simulink model "Model"  (R2023b)
settings: Solver=FixedStepAuto  StartTime=0.0  StopTime=10  FixedStep=0.002  RelTol=1e-3
model workspace (MAT data in the model file):
  a = 0
undefined symbols (not defined in the file or in its folder): X, Y, Z
libraries: sm_lib x84, nesl_utility x29, slpidlib x9, simulink x6
(part 7 of 7)

== matlab function Model/支持力结算/MATLAB Function2 ==
  data: m_w input; F_N output; T1 input; T2 input; a_w input; theta input; phi_1 input; phi_4 input; L_0 input
function F_N = fcn(m_w,T1,T2,a_w,theta,phi_1,phi_4,L_0)

l_1=0.15;
l_2=0.27;
l_3=0.27;
l_4=0.15;
l_5=0.15;g=9.80665;

J11=(2*(l_1*cos(phi_1) + (2*l_2*cos(2*atan(((4*l_2^2*(l_1*sin(phi_1) - l_4*sin(phi_4))^2 - ((l_1*sin(phi_1) - l_4*sin(phi_4))^2 + (l_5 - l_1*cos(phi_1) + l_4*cos(phi_4))^2 + l_2^2 - l_3^2)^2 + 4*l_2^2*(l_5 - l_1*cos(phi_1) + l_4*cos(phi_4))^2)^(1/2) - 2*l_2*(l_1*sin(phi_1) - l_4*sin(phi_4)))/((l_1*sin(phi_1) - l_4*sin(phi_4))^2 + (l_5 - l_1*cos(phi_1) + l_4*cos(phi_4))^2 + l_2^2 - l_3^2 + 2*l_2*(l_5 - l_1*cos(phi_1) + l_4*cos(phi_4)))))*(((8*l_1*l_2^2*cos(phi_1)*(l_1*sin(phi_1) - l_4*sin(phi_4)) - 2*(2*l_1*cos(phi_1)*(l_1*sin(phi_1) - l_4*sin(phi_4)) + 2*l_1*sin(phi_1)*(l_5 - l_1*cos(phi_1) + l_4*cos(phi_4)))*((l_1*sin(phi_1) - l_4*sin(phi_4))^2 + (l_5 - l_1*cos(phi_1) + l_4*cos(phi_4))^2 + l_2^2 - l_3^2) + 8*l_1*l_2^2*sin(phi_1)*(l_5 - l_1*cos(phi_1) + l_4*cos(phi_4)))/(2*(4*l_2^2*(l_1*sin(phi_1) - l_4*sin(phi_4))^2 - ((l_1*sin(phi_1) - l_4*sin(phi_4))^2 + (l_5 - l_1*cos(phi_1) + l_4*cos(phi_4))^2 + l_2^2 - l_3^2)^2 + 4*l_2^2*(l_5 - l_1*cos(phi_1) + l_4*cos(phi_4))^2)^(1/2)) - 2*l_1*l_2*cos(phi_1))/((l_1*sin(phi_1) - l_4*sin(phi_4))^2 + (l_5 - l_1*cos(phi_1) + l_4*cos(phi_4))^2 + l_2^2 - l_3^2 + 2*l_2*(l_5 - l_1*cos(phi_1) + l_4*cos(phi_4))) - (((4*l_2^2*(l_1*sin(phi_1) - l_4*sin(phi_4))^2 - ((l_1*sin(phi_1) - l_4*sin(phi_4))^2 + (l_5 - l_1*cos(phi_1) + l_4*cos(phi_4))^2 + l_2^2 - l_3^2)^2 + 4*l_2^2*(l_5 - l_1*cos(phi_1) + l_4*cos(phi_4))^2)^(1/2) - 2*l_2*(l_1*sin(phi_1) - l_4*sin(phi_4)))*(2*l_1*l_2*sin(phi_1) + 2*l_1*cos(phi_1)*(l_1*sin(phi_1) - l_4*sin(phi_4)) + 2*l_1*sin(phi_1)*(l_5 - l_1*cos(phi_1) + l_4*cos(phi_4))))/((l_1*sin(phi_1) - l_4*sin(phi_4))^2 + (l_5 - l_1*cos(phi_1) + l_4*cos(phi_4))^2 + l_2^2 - l_3^2 + 2*l_2*(l_5 - l_1*cos(phi_1) + l_4*cos(phi_4)))^2))/(((4*l_2^2*(l_1*sin(phi_1) - l_4*sin(phi_4))^2 - ((l_1*sin(phi_1) - l_4*sin(phi_4))^2 + (l_5 - l_1*cos(phi_1) + l_4*cos(phi_4))^2 + l_2^2 - l_3^2)^2 + 4*l_2^2*(l_5 - l_1*cos(phi_1) + l_4*cos(phi_4))^2)^(1/2) - 2*l_2*(l_1*sin(phi_1) - l_4*sin(phi_4)))^2/((l_1*sin(phi_1) - l_4*sin(phi_4))^2 + (l_5 - l_1*cos(phi_1) + l_4*cos(phi_4))^2 + l_2^2 - l_3^2 + 2*l_2*(l_5 - l_1*cos(phi_1) + l_4*cos(phi_4)))^2 + 1))*(l_2*sin(2*atan(((4*l_2^2*(l_1*sin(phi_1) - l_4*sin(phi_4))^2 - ((l_1*sin(phi_1) - l_4*sin(phi_4))^2 + (l_5 - l_1*cos(phi_1) + l_4*cos(phi_4))^2 + l_2^2 - l_3^2)^2 + 4*l_2^2*(l_5 - l_1*cos(phi_1) + l_4*cos(phi_4))^2)^(1/2) - 2*l_2*(l_1*sin(phi_1) - l_4*sin(phi_4)))/((l_1*sin(phi_1) - l_4*sin(phi_4))^2 + (l_5 - l_1*cos(phi_1) + l_4*cos(phi_4))^2 + l_2^2 - l_3^2 + 2*l_2*(l_5 - l_1*cos(phi_1) + l_4*cos(phi_4))))) + l_1*sin(phi_1)) - 2*(l_1*sin(phi_1) + (2*l_2*sin(2*atan(((4*l_2^2*(l_1*sin(phi_1) - l_4*sin(phi_4))^2 - ((l_1*sin(phi_1) - l_4*sin(phi_4))^2 + (l_5 - l_1*cos(phi_1) + l_4*cos(phi_4))^2 + l_2^2 - l_3^2)^2 + 4*l_2^2*(l_5 - l_1*cos(phi_1) + l_4*cos(phi_4))^2)^(1/2) - 2*l_2*(l_1*sin(phi_1) - l_4*sin(phi_4)))/((l_1*sin(phi_1) - l_4*sin(phi_4))^2 + (l_5 - l_1*cos(phi_1) + l_4*cos(phi_4))^2 + l_2^2 - l_3^2 + 2*l_2*(l_5 - l_1*cos(phi_1) + l_4*cos(phi_4)))))*(((8*l_1*l_2^2*cos(phi_1)*(l_1*sin(phi_1) - l_4*sin(phi_4)) - 2*(2*l_1*cos(phi_1)*(l_1*sin(phi_1) - l_4*sin(phi_4)) + 2*l_1*sin(phi_1)*(l_5 - l_1*cos(phi_1) + l_4*cos(phi_4)))*((l_1*sin(phi_1) - l_4*sin(phi_4))^2 + (l_5 - l_1*cos(phi_1) + l_4*cos(phi_4))^2 + l_2^2 - l_3^2) + 8*l_1*l_2^2*sin(phi_1)*(l_5 - l_1*cos(phi_1) + l_4*cos(phi_4)))/(2*(4*l_2^2*(l_1*sin(phi_1) - l_4*sin(phi_4))^2 - ((l_1*sin(phi_1) - l_4*sin(phi_4))^2 + (l_5 - l_1*cos(phi_1) + l_4*cos(phi_4))^2 + l_2^2 - l_3^2)^2 + 4*l_2^2*(l_5 - l_1*cos(phi_1) + l_4*cos(phi_4))^2)^(1/2)) - 2*l_1*l_2*cos(phi_1))/((l_1*sin(phi_1) - l_4*sin(phi_4))^2 + (l_5 - l_1*cos(phi_1) + l_4*cos(phi_4))^2 + l_2^2 - l_3^2 + 2*l_2*(l_5 - l_1*cos(phi_1) + l_4*cos(phi_4))) - (((4*l_2^2*(l_1*sin(phi_1) - l_4*sin(phi_4))^2 - ((l_1*sin(phi_1) - l_4*sin(phi_4))^2 + (l_5 - l_1*cos(phi_1) + l_4*cos(phi_4))^2 + l_2^2 - l_3^2)^2 + 4*l_2^2*(l_5 - l_1*cos(phi_1) + l_4*cos(phi_4))^2)^(1/2) - 2*l_2*(l_1*sin(phi_1) - l_4*sin(phi_4)))*(2*l_1*l_2*sin(phi_1) + 2*l_1*cos(phi_1)*(l_1*sin(phi_1) - l_4*sin(phi_4)) + 2*l_1*sin(phi_1)*(l_5 - l_1*cos(phi_1) + l_4*cos(phi_4))))/((l_1*sin(phi_1) - l_4*sin(phi_4))^2 + (l_5 - l_1*cos(phi_1) + l_4*cos(phi_4))^2 + l_2^2 - l_3^2 + 2*l_2*(l_5 - l_1*cos(phi_1) + l_4*cos(phi_4)))^2))/(((4*l_2^2*(l_1*sin(phi_1) - l_4*sin(phi_4))^2 - ((l_1*sin(phi_1) - l_4*sin(phi_4))^2 + (l_5 - l_1*cos(phi_1) + l_4*cos(phi_4))^2 + l_2^2 - l_3^2)^2 + 4*l_2^2*(l_5 - l_1*cos(phi_1) + l_4*cos(phi_4))^2)^(1/2) - 2*l_2*(l_1*sin(phi_1) - l_4*sin(phi_4)))^2/((l_1*sin(phi_1) - l_4*sin(phi_4))^2 + (l_5 - l_1*cos(phi_1) + l_4*cos(phi_4))^2 + l_2^2 - l_3^2 + 2*l_2*(l_5 - l_1*cos(phi_1) + l_4*cos(phi_4)))^2 + 1))*(l_2*cos(2*atan(((4*l_2^2*(l_1*sin(phi_1) - l_4*sin(phi_4))^2 - ((l_1*sin(phi_1) - l_4*sin(phi_4))^2 + (l_5 - l_1*cos(phi_1) + l_4*cos(phi_4))^2 + l_2^2 - l_3^2)^2 + 4*l_2^2*(l_5 - l_1*cos(phi_1) + l_4*cos(phi_4))^2)^(1/2) - 2*l_2*(l_1*sin(phi_1) - l_4*sin(phi_4)))/((l_1*sin(phi_1) - l_4*sin(phi_4))^2 + (l_5 - l_1*cos(phi_1) + l_4*cos(phi_4))^2 + l_2^2 - l_3^2 + 2*l_2*(l_5 - l_1*cos(phi_1) + l_4*cos(phi_4))))) - l_5/2 + l_1*cos(phi_1)))/(2*((l_2*sin(2*atan(((4*l_2^2*(l_1*sin(phi_1) - l_4*sin(phi_4))^2 - ((l_1*sin(phi_1) - l_4*sin(phi_4))^2 + (l_5 - l_1*cos(phi_1) + l_4*cos(phi_4))^2 + l_2^2 - l_3^2)^2 + 4*l_2^2*(l_5 - l_1*cos(phi_1) + l_4*cos(phi_4))^2)^(1/2) - 2*l_2*(l_1*sin(phi_1) - l_4*sin(phi_4)))/((l_1*sin(phi_1) - l_4*sin(phi_4))^2 + (l_5 - l_1*cos(phi_1) + l_4*cos(phi_4))^2 + l_2^2 - l_3^2 + 2*l_2*(l_5 - l_1*cos(phi_1) + l_4*cos(phi_4))))) + l_1*sin(phi_1))^2 + (l_2*cos(2*atan(((4*l_2^2*(l_1*sin(phi_1) - l_4*sin(phi_4))^2 - ((l_1*sin(phi_1) - l_4*sin(phi_4))^2 + (l_5 - l_1*cos(phi_1) + l_4*cos(phi_4))^2 + l_2^2 - l_3^2)^2 + 4*l_2^2*(l_5 - l_1*cos(phi_1) + l_4*cos(phi_4))^2)^(1/2) - 2*l_2*(l_1*sin(phi_1) - l_4*sin(phi_4)))/((l_1*sin(phi_1) - l_4*sin(phi_4))^2 + (l_5 - l_1*cos(phi_1) + l_4*cos(phi_4))^2 + l_2^2 - l_3^2 + 2*l_2*(l_5 - l_1*cos(phi_1) + l_4*cos(phi_4))))) - l_5/2 + l_1*cos(phi_1))^2)^(1/2));
J12=((4*l_2*sin(2*atan(((4*l_2^2*(l_1*sin(phi_1) - l_4*sin(phi_4))^2 - ((l_1*sin(phi_1) - l_4*sin(phi_4))^2 + (l_5 - l_1*cos(phi_1) + l_4*cos(phi_4))^2 + l_2^2 - l_3^2)^2 + 4*l_2^2*(l_5 - l_1*cos(phi_1) + l_4*cos(phi_4))^2)^(1/2) - 2*l_2*(l_1*sin(phi_1) - l_4*sin(phi_4)))/((l_1*sin(phi_1) - l_4*sin(phi_4))^2 + (l_5 - l_1*cos(phi_1) + l_4*cos(phi_4))^2 + l_2^2 - l_3^2 + 2*l_2*(l_5 - l_1*cos(phi_1) + l_4*cos(phi_4)))))*(((8*l_2^2*l_4*cos(phi_4)*(l_1*sin(phi_1) - l_4*sin(phi_4)) - 2*(2*l_4*cos(phi_4)*(l_1*sin(phi_1) - l_4*sin(phi_4)) + 2*l_4*sin(phi_4)*(l_5 - l_1*cos(phi_1) + l_4*cos(phi_4)))*((l_1*sin(phi_1) - l_4*sin(phi_4))^2 + (l_5 - l_1*cos(phi_1) + l_4*cos(phi_4))^2 + l_2^2 - l_3^2) + 8*l_2^2*l_4*sin(phi_4)*(l_5 - l_1*cos(phi_1) + l_4*cos(phi_4)))/(2*(4*l_2^2*(l_1*sin(phi_1) - l_4*sin(phi_4))^2 - ((l_1*sin(phi_1) - l_4*sin(phi_4))^2 + (l_5 - l_1*cos(phi_1) + l_4*cos(phi_4))^2 + l_2^2 - l_3^2)^2 + 4*l_2^2*(l_5 - l_1*cos(phi_1) + l_4*cos(phi_4))^2)^(1/2)) - 2*l_2*l_4*cos(phi_4))/((l_1*sin(phi_1) - l_4*sin(phi_4))^2 + (l_5 - l_1*cos(phi_1) + l_4*cos(phi_4))^2 + l_2^2 - l_3^2 + 2*l_2*(l_5 - l_1*cos(phi_1) + l_4*cos(phi_4))) - (((4*l_2^2*(l_1*sin(phi_1) - l_4*sin(phi_4))^2 - ((l_1*sin(phi_1) - l_4*sin(phi_4))^2 + (l_5 - l_1*cos(phi_1) + l_4*cos(phi_4))^2 + l_2^2 - l_3^2)^2 + 4*l_2^2*(l_5 - l_1*cos(phi_1) + l_4*cos(phi_4))^2)^(1/2) - 2*l_2*(l_1*sin(phi_1) - l_4*sin(phi_4)))*(2*l_2*l_4*sin(phi_4) + 2*l_4*cos(phi_4)*(l_1*sin(phi_1) - l_4*sin(phi_4)) + 2*l_4*sin(phi_4)*(l_5 - l_1*cos(phi_1) + l_4*cos(phi_4))))/((l_1*sin(phi_1) - l_4*sin(phi_4))^2 + (l_5 - l_1*cos(phi_1) + l_4*cos(phi_4))^2 + l_2^2 - l_3^2 + 2*l_2*(l_5 - l_1*cos(phi_1) + l_4*cos(phi_4)))^2)*(l_2*cos(2*atan(((4*l_2^2*(l_1*sin(phi_1) - l_4*sin(phi_4))^2 - ((l_1*sin(phi_1) - l_4*sin(phi_4))^2 + (l_5 - l_1*cos(phi_1) + l_4*cos(phi_4))^2 + l_2^2 - l_3^2)^2 + 4*l_2^2*(l_5 - l_1*cos(phi_1) + l_4*cos(phi_4))^2)^(1/2) - 2*l_2*(l_1*sin(phi_1) - l_4*sin(phi_4)))/((l_1*sin(phi_1) - l_4*sin(phi_4))^2 + (l_5 - l_1*cos(phi_1) + l_4*cos(phi_4))^2 + l_2^2 - l_3^2 + 2*l_2*(l_5 - l_1*cos(phi_1) + l_4*cos(phi_4))))) - l_5/2 + l_1*cos(phi_1)))/(((4*l_2^2*(l_1*sin(phi_1) - l_4*sin(phi_4))^2 - ((l_1*sin(phi_1) - l_4*sin(phi_4))^2 + (l_5 - l_1*cos(phi_1) + l_4*cos(phi_4))^2 + l_2^2 - l_3^2)^2 + 4*l_2^2*(l_5 - l_1*cos(phi_1) + l_4*cos(phi_4))^2)^(1/2) - 2*l_2*(l_1*sin(phi_1) - l_4*sin(phi_4)))^2/((l_1*sin(phi_1) - l_4*sin(phi_4))^2 + (l_5 - l_1*cos(phi_1) + l_4*cos(phi_4))^2 + l_2^2 - l_3^2 + 2*l_2*(l_5 - l_1*cos(phi_1) + l_4*cos(phi_4)))^2 + 1) - (4*l_2*cos(2*atan(((4*l_2^2*(l_1*sin(phi_1) - l_4*sin(phi_4))^2 - ((l_1*sin(phi_1) - l_4*sin(phi_4))^2 + (l_5 - l_1*cos(phi_1) + l_4*cos(phi_4))^2 + l_2^2 - l_3^2)^2 + 4*l_2^2*(l_5 - l_1*cos(phi_1) + l_4*cos(phi_4))^2)^(1/2) - 2*l_2*(l_1*sin(phi_1) - l_4*sin(phi_4)))/((l_1*sin(phi_1) - l_4*sin(phi_4))^2 + (l_5 - l_1*cos(phi_1) + l_4*cos(phi_4))^2 + l_2^2 - l_3^2 + 2*l_2*(l_5 - l_1*cos(phi_1) + l_4*cos(phi_4)))))*(l_2*sin(2*atan(((4*l_2^2*(l_1*sin(phi_1) - l_4*sin(phi_4))^2 - ((l_1*sin(phi_1) - l_4*sin(phi_4))^2 + (l_5 - l_1*cos(phi_1) + l_4*cos(phi_4))^2 + l_2^2 - l_3^2)^2 + 4*l_2^2*(l_5 - l_1*cos(phi_1) + l_4*cos(phi_4))^2)^(1/2) - 2*l_2*(l_1*sin(phi_1) - l_4*sin(phi_4)))/((l_1*sin(phi_1) - l_4*sin(phi_4))^2 + (l_5 - l_1*cos(phi_1) + l_4*cos(phi_4))^2 + l_2^2 - l_3^2 + 2*l_2*(l_5 - l_1*cos(phi_1) + l_4*cos(phi_4))))) + l_1*sin(phi_1))*(((8*l_2^2*l_4*cos(phi_4)*(l_1*sin(phi_1) - l_4*sin(phi_4)) - 2*(2*l_4*cos(phi_4)*(l_1*sin(phi_1) - l_4*sin(phi_4)) + 2*l_4*sin(phi_4)*(l_5 - l_1*cos(phi_1) + l_4*cos(phi_4)))*((l_1*sin(phi_1) - l_4*sin(phi_4))^2 + (l_5 - l_1*cos(phi_1) + l_4*cos(phi_4))^2 + l_2^2 - l_3^2) + 8*l_2^2*l_4*sin(phi_4)*(l_5 - l_1*cos(phi_1) + l_4*cos(phi_4)))/(2*(4*l_2^2*(l_1*sin(phi_1) - l_4*sin(phi_4))^2 - ((l_1*sin(phi_1) - l_4*sin(phi_4))^2 + (l_5 - l_1*cos(phi_1) + l_4*cos(phi_4))^2 + l_2^2 - l_3^2)^2 + 4*l_2^2*(l_5 - l_1*cos(phi_1) + l_4*cos(phi_4))^2)^(1/2)) - 2*l_2*l_4*cos(phi_4))/((l_1*sin(phi_1) - l_4*sin(phi_4))^2 + (l_5 - l_1*cos(phi_1) + l_4*cos(phi_4))^2 + l_2^2 - l_3^2 + 2*l_2*(l_5 - l_1*cos(phi_1) + l_4*cos(phi_4))) - (((4*l_2^2*(l_1*sin(phi_1) - l_4*sin(phi_4))^2 - ((l_1*sin(phi_1) - l_4*sin(phi_4))^2 + (l_5 - l_1*cos(phi_1) + l_4*cos(phi_4))^2 + l_2^2 - l_3^2)^2 + 4*l_2^2*(l_5 - l_1*cos(phi_1) + l_4*cos(phi_4))^2)^(1/2) - 2*l_2*(l_1*sin(phi_1) - l_4*sin(phi_4)))*(2*l_2*l_4*sin(phi_4) + 2*l_4*cos(phi_4)*(l_1*sin(phi_1) - l_4*sin(phi_4)) + 2*l_4*sin(phi_4)*(l_5 - l_1*cos(phi_1) + l_4*cos(phi_4))))/((l_1*sin(phi_1) - l_4*sin(phi_4))^2 + (l_5 - l_1*cos(phi_1) + l_4*cos(phi_4))^2 + l_2^2 - l_3^2 + 2*l_2*(l_5 - l_1*cos(phi_1) + l_4*cos(phi_4)))^2))/(((4*l_2^2*(l_1*sin(phi_1) - l_4*sin(phi_4))^2 - ((l_1*sin(phi_1) - l_4*sin(phi_4))^2 + (l_5 - l_1*cos(phi_1) + l_4*cos(phi_4))^2 + l_2^2 - l_3^2)^2 + 4*l_2^2*(l_5 - l_1*cos(phi_1) + l_4*cos(phi_4))^2)^(1/2) - 2*l_2*(l_1*sin(phi_1) - l_4*sin(phi_4)))^2/((l_1*sin(phi_1) - l_4*sin(phi_4))^2 + (l_5 - l_1*cos(phi_1) + l_4*cos(phi_4))^2 + l_2^2 - l_3^2 + 2*l_2*(l_5 - l_1*cos(phi_1) + l_4*cos(phi_4)))^2 + 1))/(2*((l_2*sin(2*atan(((4*l_2^2*(l_1*sin(phi_1) - l_4*sin(phi_4))^2 - ((l_1*sin(phi_1) - l_4*sin(phi_4))^2 + (l_5 - l_1*cos(phi_1) + l_4*cos(phi_4))^2 + l_2^2 - l_3^2)^2 + 4*l_2^2*(l_5 - l_1*cos(phi_1) + l_4*cos(phi_4))^2)^(1/2) - 2*l_2*(l_1*sin(phi_1) - l_4*sin(phi_4)))/((l_1*sin(phi_1) - l_4*sin(phi_4))^2 + (l_5 - l_1*cos(phi_1) + l_4*cos(phi_4))^2 + l_2^2 - l_3^2 + 2*l_2*(l_5 - l_1*cos(phi_1) + l_4*cos(phi_4))))) + l_1*sin(phi_1))^2 + (l_2*cos(2*atan(((4*l_2^2*(l_1*sin(phi_1) - l_4*sin(phi_4))^2 - ((l_1*sin(phi_1) - l_4*sin(phi_4))^2 + (l_5 - l_1*cos(phi_1) + l_4*cos(phi_4))^2 + l_2^2 - l_3^2)^2 + 4*l_2^2*(l_5 - l_1*cos(phi_1) + l_4*cos(phi_4))^2)^(1/2) - 2*l_2*(l_1*sin(phi_1) - l_4*sin(phi_4)))/((l_1*sin(phi_1) - l_4*sin(phi_4))^2 + (l_5 - l_1*cos(phi_1) + l_4*cos(phi_4))^2 + l_2^2 - l_3^2 + 2*l_2*(l_5 - l_1*cos(phi_1) + l_4*cos(phi_4))))) - l_5/2 + l_1*cos(phi_1))^2)^(1/2));
J21=((l_1*sin(phi_1) + (2*l_2*sin(2*atan(((4*l_2^2*(l_1*sin(phi_1) - l_4*sin(phi_4))^2 - ((l_1*sin(phi_1) - l_4*sin(phi_4))^2 + (l_5 - l_1*cos(phi_1) + l_4*cos(phi_4))^2 + l_2^2 - l_3^2)^2 + 4*l_2^2*(l_5 - l_1*cos(phi_1) + l_4*cos(phi_4))^2)^(1/2) - 2*l_2*(l_1*sin(phi_1) - l_4*sin(phi_4)))/((l_1*sin(phi_1) - l_4*sin(phi_4))^2 + (l_5 - l_1*cos(phi_1) + l_4*cos(phi_4))^2 + l_2^2 - l_3^2 + 2*l_2*(l_5 - l_1*cos(phi_1) + l_4*cos(phi_4)))))*(((8*l_1*l_2^2*cos(phi_1)*(l_1*sin(phi_1) - l_4*sin(phi_4)) - 2*(2*l_1*cos(phi_1)*(l_1*sin(phi_1) - l_4*sin(phi_4)) + 2*l_1*sin(phi_1)*(l_5 - l_1*cos(phi_1) + l_4*cos(phi_4)))*((l_1*sin(phi_1) - l_4*sin(phi_4))^2 + (l_5 - l_1*cos(phi_1) + l_4*cos(phi_4))^2 + l_2^2 - l_3^2) + 8*l_1*l_2^2*sin(phi_1)*(l_5 - l_1*cos(phi_1) + l_4*cos(phi_4)))/(2*(4*l_2^2*(l_1*sin(phi_1) - l_4*sin(phi_4))^2 - ((l_1*sin(phi_1) - l_4*sin(phi_4))^2 + (l_5 - l_1*cos(phi_1) + l_4*cos(phi_4))^2 + l_2^2 - l_3^2)^2 + 4*l_2^2*(l_5 - l_1*cos(phi_1) + l_4*cos(phi_4))^2)^(1/2)) - 2*l_1*l_2*cos(phi_1))/((l_1*sin(phi_1) - l_4*sin(phi_4))^2 + (l_5 - l_1*cos(phi_1) + l_4*cos(phi_4))^2 + l_2^2 - l_3^2 + 2*l_2*(l_5 - l_1*cos(phi_1) + l_4*cos(phi_4))) - (((4*l_2^2*(l_1*sin(phi_1) - l_4*sin(phi_4))^2 - ((l_1*sin(phi_1) - l_4*sin(phi_4))^2 + (l_5 - l_1*cos(phi_1) + l_4*cos(phi_4))^2 + l_2^2 - l_3^2)^2 + 4*l_2^2*(l_5 - l_1*cos(phi_1) + l_4*cos(phi_4))^2)^(1/2) - 2*l_2*(l_1*sin(phi_1) - l_4*sin(phi_4)))*(2*l_1*l_2*sin(phi_1) + 2*l_1*cos(phi_1)*(l_1*sin(phi_1) - l_4*sin(phi_4)) + 2*l_1*sin(phi_1)*(l_5 - l_1*cos(phi_1) + l_4*cos(phi_4))))/((l_1*sin(phi_1) - l_4*sin(phi_4))^2 + (l_5 - l_1*cos(phi_1) + l_4*cos(phi_4))^2 + l_2^2 - l_3^2 + 2*l_2*(l_5 - l_1*cos(phi_1) + l_4*cos(phi_4)))^2))/(((4*l_2^2*(l_1*sin(phi_1) - l_4*sin(phi_4))^2 - ((l_1*sin(phi_1) - l_4*sin(phi_4))^2 + (l_5 - l_1*cos(phi_1) + l_4*cos(phi_4))^2 + l_2^2 - l_3^2)^2 + 4*l_2^2*(l_5 - l_1*cos(phi_1) + l_4*cos(phi_4))^2)^(1/2) - 2*l_2*(l_1*sin(phi_1) - l_4*sin(phi_4)))^2/((l_1*sin(phi_1) - l_4*sin(phi_4))^2 + (l_5 - l_1*cos(phi_1) + l_4*cos(phi_4))^2 + l_2^2 - l_3^2 + 2*l_2*(l_5 - l_1*cos(phi_1) + l_4*cos(phi_4)))^2 + 1))/((l_2*sin(2*atan(((4*l_2^2*(l_1*sin(phi_1) - l_4*sin(phi_4))^2 - ((l_1*sin(phi_1) - l_4*sin(phi_4))^2 + (l_5 - l_1*cos(phi_1) + l_4*cos(phi_4))^2 + l_2^2 - l_3^2)^2 + 4*l_2^2*(l_5 - l_1*cos(phi_1) + l_4*cos(phi_4))^2)^(1/2) - 2*l_2*(l_1*sin(phi_1) - l_4*sin(phi_4)))/((l_1*sin(phi_1) - l_4*sin(phi_4))^2 + (l_5 - l_1*cos(phi_1) + l_4*cos(phi_4))^2 + l_2^2 - l_3^2 + 2*l_2*(l_5 - l_1*cos(phi_1) + l_4*cos(phi_4))))) + l_1*sin(phi_1))^2 + (l_2*cos(2*atan(((4*l_2^2*(l_1*sin(phi_1) - l_4*sin(phi_4))^2 - ((l_1*sin(phi_1) - l_4*sin(phi_4))^2 + (l_5 - l_1*cos(phi_1) + l_4*cos(phi_4))^2 + l_2^2 - l_3^2)^2 + 4*l_2^2*(l_5 - l_1*cos(phi_1) + l_4*cos(phi_4))^2)^(1/2) - 2*l_2*(l_1*sin(phi_1) - l_4*sin(phi_4)))/((l_1*sin(phi_1) - l_4*sin(phi_4))^2 + (l_5 - l_1*cos(phi_1) + l_4*cos(phi_4))^2 + l_2^2 - l_3^2 + 2*l_2*(l_5 - l_1*cos(phi_1) + l_4*cos(phi_4))))) - l_5/2 + l_1*cos(phi_1))^2)^(1/2) + ((2*(l_1*cos(phi_1) + (2*l_2*cos(2*atan(((4*l_2^2*(l_1*sin(phi_1) - l_4*sin(phi_4))^2 - ((l_1*sin(phi_1) - l_4*sin(phi_4))^2 + (l_5 - l_1*cos(phi_1) + l_4*cos(phi_4))^2 + l_2^2 - l_3^2)^2 + 4*l_2^2*(l_5 - l_1*cos(phi_1) + l_4*cos(phi_4))^2)^(1/2) - 2*l_2*(l_1*sin(phi_1) - l_4*sin(phi_4)))/((l_1*sin(phi_1) - l_4*sin(phi_4))^2 + (l_5 - l_1*cos(phi_1) + l_4*cos(phi_4))^2 + l_2^2 - l_3^2 + 2*l_2*(l_5 - l_1*cos(phi_1) + l_4*cos(phi_4)))))*(((8*l_1*l_2^2*cos(phi_1)*(l_1*sin(phi_1) - l_4*sin(phi_4)) - 2*(2*l_1*cos(phi_1)*(l_1*sin(phi_1) - l_4*sin(phi_4)) + 2*l_1*sin(phi_1)*(l_5 - l_1*cos(phi_1) + l_4*cos(phi_4)))*((l_1*sin(phi_1) - l_4*sin(phi_4))^2 + (l_5 - l_1*cos(phi_1) + l_4*cos(phi_4))^2 + l_2^2 - l_3^2) + 8*l_1*l_2^2*sin(phi_1)*(l_5 - l_1*cos(phi_1) + l_4*cos(phi_4)))/(2*(4*l_2^2*(l_1*sin(phi_1) - l_4*sin(phi_4))^2 - ((l_1*sin(phi_1) - l_4*sin(phi_4))^2 + (l_5 - l_1*cos(phi_1) + l_4*cos(phi_4))^2 + l_2^2 - l_3^2)^2 + 4*l_2^2*(l_5 - l_1*cos(phi_1) + l_4*cos(phi_4))^2)^(1/2)) - 2*l_1*l_2*cos(phi_1))/((l_1*sin(phi_1) - l_4*sin(phi_4))^2 + (l_5 - l_1*cos(phi_1) + l_4*cos(phi_4))^2 + l_2^2 - l_3^2 + 2*l_2*(l_5 - l_1*cos(phi_1) + l_4*cos(phi_4))) - (((4*l_2^2*(l_1*sin(phi_1) - l_4*sin(phi_4))^2 - ((l_1*sin(phi_1) - l_4*sin(phi_4))^2 + (l_5 - l_1*cos(phi_1) + l_4*cos(phi_4))^2 + l_2^2 - l_3^2)^2 + 4*l_2^2*(l_5 - l_1*cos(phi_1) + l_4*cos(phi_4))^2)^(1/2) - 2*l_2*(l_1*sin(phi_1) - l_4*sin(phi_4)))*(2*l_1*l_2*sin(phi_1) + 2*l_1*cos(phi_1)*(l_1*sin(phi_1) - l_4*sin(phi_4)) + 2*l_1*sin(phi_1)*(l_5 - l_1*cos(phi_1) + l_4*cos(phi_4))))/((l_1*sin(phi_1) - l_4*sin(phi_4))^2 + (l_5 - l_1*cos(phi_1) + l_4*cos(phi_4))^2 + l_2^2 - l_3^2 + 2*l_2*(l_5 - l_1*cos(phi_1) + l_4*cos(phi_4)))^2))/(((4*l_2^2*(l_1*sin(phi_1) - l_4*sin(phi_4))^2 - ((l_1*sin(phi_1) - l_4*sin(phi_4))^2 + (l_5 - l_1*cos(phi_1) + l_4*cos(phi_4))^2 + l_2^2 - l_3^2)^2 + 4*l_2^2*(l_5 - l_1*cos(phi_1) + l_4*cos(phi_4))^2)^(1/2) - 2*l_2*(l_1*sin(phi_1) - l_4*sin(phi_4)))^2/((l_1*sin(phi_1) - l_4*sin(phi_4))^2 + (l_5 - l_1*cos(phi_1) + l_4*cos(phi_4))^2 + l_2^2 - l_3^2 + 2*l_2*(l_5 - l_1*cos(phi_1) + l_4*cos(phi_4)))^2 + 1))*(l_2*sin(2*atan(((4*l_2^2*(l_1*sin(phi_1) - l_4*sin(phi_4))^2 - ((l_1*sin(phi_1) - l_4*sin(phi_4))^2 + (l_5 - l_1*cos(phi_1) + l_4*cos(phi_4))^2 + l_2^2 - l_3^2)^2 + 4*l_2^2*(l_5 - l_1*cos(phi_1) + l_4*cos(phi_4))^2)^(1/2) - 2*l_2*(l_1*sin(phi_1) - l_4*sin(phi_4)))/((l_1*sin(phi_1) - l_4*sin(phi_4))^2 + (l_5 - l_1*cos(phi_1) + l_4*cos(phi_4))^2 + l_2^2 - l_3^2 + 2*l_2*(l_5 - l_1*cos(phi_1) + l_4*cos(phi_4))))) + l_1*sin(phi_1)) - 2*(l_1*sin(phi_1) + (2*l_2*sin(2*atan(((4*l_2^2*(l_1*sin(phi_1) - l_4*sin(phi_4))^2 - ((l_1*sin(phi_1) - l_4*sin(phi_4))^2 + (l_5 - l_1*cos(phi_1) + l_4*cos(phi_4))^2 + l_2^2 - l_3^2)^2 + 4*l_2^2*(l_5 - l_1*cos(phi_1) + l_4*cos(phi_4))^2)^(1/2) - 2*l_2*(l_1*sin(phi_1) - l_4*sin(phi_4)))/((l_1*sin(phi_1) - l_4*sin(phi_4))^2 + (l_5 - l_1*cos(phi_1) + l_4*cos(phi_4))^2 + l_2^2 - l_3^2 + 2*l_2*(l_5 - l_1*cos(phi_1) + l_4*cos(phi_4)))))*(((8*l_1*l_2^2*cos(phi_1)*(l_1*sin(phi_1) - l_4*sin(phi_4)) - 2*(2*l_1*cos(phi_1)*(l_1*sin(phi_1) - l_4*sin(phi_4)) + 2*l_1*sin(phi_1)*(l_5 - l_1*cos(phi_1) + l_4*cos(phi_4)))*((l_1*sin(phi_1) - l_4*sin(phi_4))^2 + (l_5 - l_1*cos(phi_1) + l_4*cos(phi_4))^2 + l_2^2 - l_3^2) + 8*l_1*l_2^2*sin(phi_1)*(l_5 - l_1*cos(phi_1) + l_4*cos(phi_4)))/(2*(4*l_2^2*(l_1*sin(phi_1) - l_4*sin(phi_4))^2 - ((l_1*sin(phi_1) - l_4*sin(phi_4))^2 + (l_5 - l_1*cos(phi_1) + l_4*cos(phi_4))^2 + l_2^2 - l_3^2)^2 + 4*l_2^2*(l_5 - l_1*cos(phi_1) + l_4*cos(phi_4))^2)^(1/2)) - 2*l_1*l_2*cos(phi_1))/((l_1*sin(phi_1) - l_4*sin(phi_4))^2 + (l_5 - l_1*cos(phi_1) + l_4*cos(phi_4))^2 + l_2^2 - l_3^2 + 2*l_2*(l_5 - l_1*cos(phi_1) + l_4*cos(phi_4))) - (((4*l_2^2*(l_1*sin(phi_1) - l_4*sin(phi_4))^2 - ((l_1*sin(phi_1) - l_4*sin(phi_4))^2 + (l_5 - l_1*cos(phi_1) + l_4*cos(phi_4))^2 + l_2^2 - l_3^2)^2 + 4*l_2^2*(l_5 - l_1*cos(phi_1) + l_4*cos(phi_4))^2)^(1/2) - 2*l_2*(l_1*sin(phi_1) - l_4*sin(phi_4)))*(2*l_1*l_2*sin(phi_1) + 2*l_1*cos(phi_1)*(l_1*sin(phi_1) - l_4*sin(phi_4)) + 2*l_1*sin(phi_1)*(l_5 - l_1*cos(phi_1) + l_4*cos(phi_4))))/((l_1*sin(phi_1) - l_4*sin(phi_4))^2 + (l_5 - l_1*cos(phi_1) + l_4*cos(phi_4))^2 + l_2^2 - l_3^2 + 2*l_2*(l_5 - l_1*cos(phi_1) + l_4*cos(phi_4)))^2))/(((4*l_2^2*(l_1*sin(phi_1) - l_4*sin(phi_4))^2 - ((l_1*sin(phi_1) - l_4*sin(phi_4))^2 + (l_5 - l_1*cos(phi_1) + l_4*cos(phi_4))^2 + l_2^2 - l_3^2)^2 + 4*l_2^2*(l_5 - l_1*cos(phi_1) + l_4*cos(phi_4))^2)^(1/2) - 2*l_2*(l_1*sin(phi_1) - l_4*sin(phi_4)))^2/((l_1*sin(phi_1) - l_4*sin(phi_4))^2 + (l_5 - l_1*cos(phi_1) + l_4*cos(phi_4))^2 + l_2^2 - l_3^2 + 2*l_2*(l_5 - l_1*cos(phi_1) + l_4*cos(phi_4)))^2 + 1))*(l_2*cos(2*atan(((4*l_2^2*(l_1*sin(phi_1) - l_4*sin(phi_4))^2 - ((l_1*sin(phi_1) - l_4*sin(phi_4))^2 + (l_5 - l_1*cos(phi_1) + l_4*cos(phi_4))^2 + l_2^2 - l_3^2)^2 + 4*l_2^2*(l_5 - l_1*cos(phi_1) + l_4*cos(phi_4))^2)^(1/2) - 2*l_2*(l_1*sin(phi_1) - l_4*sin(phi_4)))/((l_1*sin(phi_1) - l_4*sin(phi_4))^2 + (l_5 - l_1*cos(phi_1) + l_4*cos(phi_4))^2 + l_2^2 - l_3^2 + 2*l_2*(l_5 - l_1*cos(phi_1) + l_4*cos(phi_4))))) - l_5/2 + l_1*cos(phi_1)))*(l_2*cos(2*atan(((4*l_2^2*(l_1*sin(phi_1) - l_4*sin(phi_4))^2 - ((l_1*sin(phi_1) - l_4*sin(phi_4))^2 + (l_5 - l_1*cos(phi_1) + l_4*cos(phi_4))^2 + l_2^2 - l_3^2)^2 + 4*l_2^2*(l_5 - l_1*cos(phi_1) + l_4*cos(phi_4))^2)^(1/2) - 2*l_2*(l_1*sin(phi_1) - l_4*sin(phi_4)))/((l_1*sin(phi_1) - l_4*sin(phi_4))^2 + (l_5 - l_1*cos(phi_1) + l_4*cos(phi_4))^2 + l_2^2 - l_3^2 + 2*l_2*(l_5 - l_1*cos(phi_1) + l_4*cos(phi_4))))) - l_5/2 + l_1*cos(phi_1)))/(2*((l_2*sin(2*atan(((4*l_2^2*(l_1*sin(phi_1) - l_4*sin(phi_4))^2 - ((l_1*sin(phi_1) - l_4*sin(phi_4))^2 + (l_5 - l_1*cos(phi_1) + l_4*cos(phi_4))^2 + l_2^2 - l_3^2)^2 + 4*l_2^2*(l_5 - l_1*cos(phi_1) + l_4*cos(phi_4))^2)^(1/2) - 2*l_2*(l_1*sin(phi_1) - l_4*sin(phi_4)))/((l_1*sin(phi_1) - l_4*sin(phi_4))^2 + (l_5 - l_1*cos(phi_1) + l_4*cos(phi_4))^2 + l_2^2 - l_3^2 + 2*l_2*(l_5 - l_1*cos(phi_1) + l_4*cos(phi_4))))) + l_1*sin(phi_1))^2 + (l_2*cos(2*atan(((4*l_2^2*(l_1*sin(phi_1) - l_4*sin(phi_4))^2 - ((l_1*sin(phi_1) - l_4*sin(phi_4))^2 + (l_5 - l_1*cos(phi_1) + l_4*cos(phi_4))^2 + l_2^2 - l_3^2)^2 + 4*l_2^2*(l_5 - l_1*cos(phi_1) + l_4*cos(phi_4))^2)^(1/2) - 2*l_2*(l_1*sin(phi_1) - l_4*sin(phi_4)))/((l_1*sin(phi_1) - l_4*sin(phi_4))^2 + (l_5 - l_1*cos(phi_1) + l_4*cos(phi_4))^2 + l_2^2 - l_3^2 + 2*l_2*(l_5 - l_1*cos(phi_1) + l_4*cos(phi_4))))) - l_5/2 + l_1*cos(phi_1))^2)^(3/2)))/(1 - (l_2*cos(2*atan(((4*l_2^2*(l_1*sin(phi_1) - l_4*sin(phi_4))^2 - ((l_1*sin(phi_1) - l_4*sin(phi_4))^2 + (l_5 - l_1*cos(phi_1) + l_4*cos(phi_4))^2 + l_2^2 - l_3^2)^2 + 4*l_2^2*(l_5 - l_1*cos(phi_1) + l_4*cos(phi_4))^2)^(1/2) - 2*l_2*(l_1*sin(phi_1) - l_4*sin(phi_4)))/((l_1*sin(phi_1) - l_4*sin(phi_4))^2 + (l_5 - l_1*cos(phi_1) + l_4*cos(phi_4))^2 + l_2^2 - l_3^2 + 2*l_2*(l_5 - l_1*cos(phi_1) + l_4*cos(phi_4))))) - l_5/2 + l_1*cos(phi_1))^2/((l_2*sin(2*atan(((4*l_2^2*(l_1*sin(phi_1) - l_4*sin(phi_4))^2 - ((l_1*sin(phi_1) - l_4*sin(phi_4))^2 + (l_5 - l_1*cos(phi_1) + l_4*cos(phi_4))^2 + l_2^2 - l_3^2)^2 + 4*l_2^2*(l_5 - l_1*cos(phi_1) + l_4*cos(phi_4))^2)^(1/2) - 2*l_2*(l_1*sin(phi_1) - l_4*sin(phi_4)))/((l_1*sin(phi_1) - l_4*sin(phi_4))^2 + (l_5 - l_1*cos(phi_1) + l_4*cos(phi_4))^2 + l_2^2 - l_3^2 + 2*l_2*(l_5 - l_1*cos(phi_1) + l_4*cos(phi_4))))) + l_1*sin(phi_1))^2 + (l_2*cos(2*atan(((4*l_2^2*(l_1*sin(phi_1) - l_4*sin(phi_4))^2 - ((l_1*sin(phi_1) - l_4*sin(phi_4))^2 + (l_5 - l_1*cos(phi_1) + l_4*cos(phi_4))^2 + l_2^2 - l_3^2)^2 + 4*l_2^2*(l_5 - l_1*cos(phi_1) + l_4*cos(phi_4))^2)^(1/2) - 2*l_2*(l_1*sin(phi_1) - l_4*sin(phi_4)))/((l_1*sin(phi_1) - l_4*sin(phi_4))^2 + (l_5 - l_1*cos(phi_1) + l_4*cos(phi_4))^2 + l_2^2 - l_3^2 + 2*l_2*(l_5 - l_1*cos(phi_1) + l_4*cos(phi_4))))) - l_5/2 + l_1*cos(phi_1))^2))^(1/2);
J22=((((4*l_2*sin(2*atan(((4*l_2^2*(l_1*sin(phi_1) - l_4*sin(phi_4))^2 - ((l_1*sin(phi_1) - l_4*sin(phi_4))^2 + (l_5 - l_1*cos(phi_1) + l_4*cos(phi_4))^2 + l_2^2 - l_3^2)^2 + 4*l_2^2*(l_5 - l_1*cos(phi_1) + l_4*cos(phi_4))^2)^(1/2) - 2*l_2*(l_1*sin(phi_1) - l_4*sin(phi_4)))/((l_1*sin(phi_1) - l_4*sin(phi_4))^2 + (l_5 - l_1*cos(phi_1) + l_4*cos(phi_4))^2 + l_2^2 - l_3^2 + 2*l_2*(l_5 - l_1*cos(phi_1) + l_4*cos(phi_4)))))*(((8*l_2^2*l_4*cos(phi_4)*(l_1*sin(phi_1) - l_4*sin(phi_4)) - 2*(2*l_4*cos(phi_4)*(l_1*sin(phi_1) - l_4*sin(phi_4)) + 2*l_4*sin(phi_4)*(l_5 - l_1*cos(phi_1) + l_4*cos(phi_4)))*((l_1*sin(phi_1) - l_4*sin(phi_4))^2 + (l_5 - l_1*cos(phi_1) + l_4*cos(phi_4))^2 + l_2^2 - l_3^2) + 8*l_2^2*l_4*sin(phi_4)*(l_5 - l_1*cos(phi_1) + l_4*cos(phi_4)))/(2*(4*l_2^2*(l_1*sin(phi_1) - l_4*sin(phi_4))^2 - ((l_1*sin(phi_1) - l_4*sin(phi_4))^2 + (l_5 - l_1*cos(phi_1) + l_4*cos(phi_4))^2 + l_2^2 - l_3^2)^2 + 4*l_2^2*(l_5 - l_1*cos(phi_1) + l_4*cos(phi_4))^2)^(1/2)) - 2*l_2*l_4*cos(phi_4))/((l_1*sin(phi_1) - l_4*sin(phi_4))^2 + (l_5 - l_1*cos(phi_1) + l_4*cos(phi_4))^2 + l_2^2 - l_3^2 + 2*l_2*(l_5 - l_1*cos(phi_1) + l_4*cos(phi_4))) - (((4*l_2^2*(l_1*sin(phi_1) - l_4*sin(phi_4))^2 - ((l_1*sin(phi_1) - l_4*sin(phi_4))^2 + (l_5 - l_1*cos(phi_1) + l_4*cos(phi_4))^2 + l_2^2 - l_3^2)^2 + 4*l_2^2*(l_5 - l_1*cos(phi_1) + l_4*cos(phi_4))^2)^(1/2) - 2*l_2*(l_1*sin(phi_1) - l_4*sin(phi_4)))*(2*l_2*l_4*sin(phi_4) + 2*l_4*cos(phi_4)*(l_1*sin(phi_1) - l_4*sin(phi_4)) + 2*l_4*sin(phi_4)*(l_5 - l_1*cos(phi_1) + l_4*cos(phi_4))))/((l_1*sin(phi_1) - l_4*sin(phi_4))^2 + (l_5 - l_1*cos(phi_1) + l_4*cos(phi_4))^2 + l_2^2 - l_3^2 + 2*l_2*(l_5 - l_1*cos(phi_1) + l_4*cos(phi_4)))^2)*(l_2*cos(2*atan(((4*l_2^2*(l_1*sin(phi_1) - l_4*sin(phi_4))^2 - ((l_1*sin(phi_1) - l_4*sin(phi_4))^2 + (l_5 - l_1*cos(phi_1) + l_4*cos(phi_4))^2 + l_2^2 - l_3^2)^2 + 4*l_2^2*(l_5 - l_1*cos(phi_1) + l_4*cos(phi_4))^2)^(1/2) - 2*l_2*(l_1*sin(phi_1) - l_4*sin(phi_4)))/((l_1*sin(phi_1) - l_4*sin(phi_4))^2 + (l_5 - l_1*cos(phi_1) + l_4*cos(phi_4))^2 + l_2^2 - l_3^2 + 2*l_2*(l_5 - l_1*cos(phi_1) + l_4*cos(phi_4))))) - l_5/2 + l_1*cos(phi_1)))/(((4*l_2^2*(l_1*sin(phi_1) - l_4*sin(phi_4))^2 - ((l_1*sin(phi_1) - l_4*sin(phi_4))^2 + (l_5 - l_1*cos(phi_1) + l_4*cos(phi_4))^2 + l_2^2 - l_3^2)^2 + 4*l_2^2*(l_5 - l_1*cos(phi_1) + l_4*cos(phi_4))^2)^(1/2) - 2*l_2*(l_1*sin(phi_1) - l_4*sin(phi_4)))^2/((l_1*sin(phi_1) - l_4*sin(phi_4))^2 + (l_5 - l_1*cos(phi_1) + l_4*cos(phi_4))^2 + l_2^2 - l_3^2 + 2*l_2*(l_5 - l_1*cos(phi_1) + l_4*cos(phi_4)))^2 + 1) - (4*l_2*cos(2*atan(((4*l_2^2*(l_1*sin(phi_1) - l_4*sin(phi_4))^2 - ((l_1*sin(phi_1) - l_4*sin(phi_4))^2 + (l_5 - l_1*cos(phi_1) + l_4*cos(phi_4))^2 + l_2^2 - l_3^2)^2 + 4*l_2^2*(l_5 - l_1*cos(phi_1) + l_4*cos(phi_4))^2)^(1/2) - 2*l_2*(l_1*sin(phi_1) - l_4*sin(phi_4)))/((l_1*sin(phi_1) - l_4*sin(phi_4))^2 + (l_5 - l_1*cos(phi_1) + l_4*cos(phi_4))^2 + l_2^2 - l_3^2 + 2*l_2*(l_5 - l_1*cos(phi_1) + l_4*cos(phi_4)))))*(l_2*sin(2*atan(((4*l_2^2*(l_1*sin(phi_1) - l_4*sin(phi_4))^2 - ((l_1*sin(phi_1) - l_4*sin(phi_4))^2 + (l_5 - l_1*cos(phi_1) + l_4*cos(phi_4))^2 + l_2^2 - l_3^2)^2 + 4*l_2^2*(l_5 - l_1*cos(phi_1) + l_4*cos(phi_4))^2)^(1/2) - 2*l_2*(l_1*sin(phi_1) - l_4*sin(phi_4)))/((l_1*sin(phi_1) - l_4*sin(phi_4))^2 + (l_5 - l_1*cos(phi_1) + l_4*cos(phi_4))^2 + l_2^2 - l_3^2 + 2*l_2*(l_5 - l_1*cos(phi_1) + l_4*cos(phi_4))))) + l_1*sin(phi_1))*(((8*l_2^2*l_4*cos(phi_4)*(l_1*sin(phi_1) - l_4*sin(phi_4)) - 2*(2*l_4*cos(phi_4)*(l_1*sin(phi_1) - l_4*sin(phi_4)) + 2*l_4*sin(phi_4)*(l_5 - l_1*cos(phi_1) + l_4*cos(phi_4)))*((l_1*sin(phi_1) - l_4*sin(phi_4))^2 + (l_5 - l_1*cos(phi_1) + l_4*cos(phi_4))^2 + l_2^2 - l_3^2) + 8*l_2^2*l_4*sin(phi_4)*(l_5 - l_1*cos(phi_1) + l_4*cos(phi_4)))/(2*(4*l_2^2*(l_1*sin(phi_1) - l_4*sin(phi_4))^2 - ((l_1*sin(phi_1) - l_4*sin(phi_4))^2 + (l_5 - l_1*cos(phi_1) + l_4*cos(phi_4))^2 + l_2^2 - l_3^2)^2 + 4*l_2^2*(l_5 - l_1*cos(phi_1) + l_4*cos(phi_4))^2)^(1/2)) - 2*l_2*l_4*cos(phi_4))/((l_1*sin(phi_1) - l_4*sin(phi_4))^2 + (l_5 - l_1*cos(phi_1) + l_4*cos(phi_4))^2 + l_2^2 - l_3^2 + 2*l_2*(l_5 - l_1*cos(phi_1) + l_4*cos(phi_4))) - (((4*l_2^2*(l_1*sin(phi_1) - l_4*sin(phi_4))^2 - ((l_1*sin(phi_1) - l_4*sin(phi_4))^2 + (l_5 - l_1*cos(phi_1) + l_4*cos(phi_4))^2 + l_2^2 - l_3^2)^2 + 4*l_2^2*(l_5 - l_1*cos(phi_1) + l_4*cos(phi_4))^2)^(1/2) - 2*l_2*(l_1*sin(phi_1) - l_4*sin(phi_4)))*(2*l_2*l_4*sin(phi_4) + 2*l_4*cos(phi_4)*(l_1*sin(phi_1) - l_4*sin(phi_4)) + 2*l_4*sin(phi_4)*(l_5 - l_1*cos(phi_1) + l_4*cos(phi_4))))/((l_1*sin(phi_1) - l_4*sin(phi_4))^2 + (l_5 - l_1*cos(phi_1) + l_4*cos(phi_4))^2 + l_2^2 - l_3^2 + 2*l_2*(l_5 - l_1*cos(phi_1) + l_4*cos(phi_4)))^2))/(((4*l_2^2*(l_1*sin(phi_1) - l_4*sin(phi_4))^2 - ((l_1*sin(phi_1) - l_4*sin(phi_4))^2 + (l_5 - l_1*cos(phi_1) + l_4*cos(phi_4))^2 + l_2^2 - l_3^2)^2 + 4*l_2^2*(l_5 - l_1*cos(phi_1) + l_4*cos(phi_4))^2)^(1/2) - 2*l_2*(l_1*sin(phi_1) - l_4*sin(phi_4)))^2/((l_1*sin(phi_1) - l_4*sin(phi_4))^2 + (l_5 - l_1*cos(phi_1) + l_4*cos(phi_4))^2 + l_2^2 - l_3^2 + 2*l_2*(l_5 - l_1*cos(phi_1) + l_4*cos(phi_4)))^2 + 1))*(l_2*cos(2*atan(((4*l_2^2*(l_1*sin(phi_1) - l_4*sin(phi_4))^2 - ((l_1*sin(phi_1) - l_4*sin(phi_4))^2 + (l_5 - l_1*cos(phi_1) + l_4*cos(phi_4))^2 + l_2^2 - l_3^2)^2 + 4*l_2^2*(l_5 - l_1*cos(phi_1) + l_4*cos(phi_4))^2)^(1/2) - 2*l_2*(l_1*sin(phi_1) - l_4*sin(phi_4)))/((l_1*sin(phi_1) - l_4*sin(phi_4))^2 + (l_5 - l_1*cos(phi_1) + l_4*cos(phi_4))^2 + l_2^2 - l_3^2 + 2*l_2*(l_5 - l_1*cos(phi_1) + l_4*cos(phi_4))))) - l_5/2 + l_1*cos(phi_1)))/(2*((l_2*sin(2*atan(((4*l_2^2*(l_1*sin(phi_1) - l_4*sin(phi_4))^2 - ((l_1*sin(phi_1) - l_4*sin(phi_4))^2 + (l_5 - l_1*cos(phi_1) + l_4*cos(phi_4))^2 + l_2^2 - l_3^2)^2 + 4*l_2^2*(l_5 - l_1*cos(phi_1) + l_4*cos(phi_4))^2)^(1/2) - 2*l_2*(l_1*sin(phi_1) - l_4*sin(phi_4)))/((l_1*sin(phi_1) - l_4*sin(phi_4))^2 + (l_5 - l_1*cos(phi_1) + l_4*cos(phi_4))^2 + l_2^2 - l_3^2 + 2*l_2*(l_5 - l_1*cos(phi_1) + l_4*cos(phi_4))))) + l_1*sin(phi_1))^2 + (l_2*cos(2*atan(((4*l_2^2*(l_1*sin(phi_1) - l_4*sin(phi_4))^2 - ((l_1*sin(phi_1) - l_4*sin(phi_4))^2 + (l_5 - l_1*cos(phi_1) + l_4*cos(phi_4))^2 + l_2^2 - l_3^2)^2 + 4*l_2^2*(l_5 - l_1*cos(phi_1) + l_4*cos(phi_4))^2)^(1/2) - 2*l_2*(l_1*sin(phi_1) - l_4*sin(phi_4)))/((l_1*sin(phi_1) - l_4*sin(phi_4))^2 + (l_5 - l_1*cos(phi_1) + l_4*cos(phi_4))^2 + l_2^2 - l_3^2 + 2*l_2*(l_5 - l_1*cos(phi_1) + l_4*cos(phi_4))))) - l_5/2 + l_1*cos(phi_1))^2)^(3/2)) - (2*l_2*sin(2*atan(((4*l_2^2*(l_1*sin(phi_1) - l_4*sin(phi_4))^2 - ((l_1*sin(phi_1) - l_4*sin(phi_4))^2 + (l_5 - l_1*cos(phi_1) + l_4*cos(phi_4))^2 + l_2^2 - l_3^2)^2 + 4*l_2^2*(l_5 - l_1*cos(phi_1) + l_4*cos(phi_4))^2)^(1/2) - 2*l_2*(l_1*sin(phi_1) - l_4*sin(phi_4)))/((l_1*sin(phi_1) - l_4*sin(phi_4))^2 + (l_5 - l_1*cos(phi_1) + l_4*cos(phi_4))^2 + l_2^2 - l_3^2 + 2*l_2*(l_5 - l_1*cos(phi_1) + l_4*cos(phi_4)))))*(((8*l_2^2*l_4*cos(phi_4)*(l_1*sin(phi_1) - l_4*sin(phi_4)) - 2*(2*l_4*cos(phi_4)*(l_1*sin(phi_1) - l_4*sin(phi_4)) + 2*l_4*sin(phi_4)*(l_5 - l_1*cos(phi_1) + l_4*cos(phi_4)))*((l_1*sin(phi_1) - l_4*sin(phi_4))^2 + (l_5 - l_1*cos(phi_1) + l_4*cos(phi_4))^2 + l_2^2 - l_3^2) + 8*l_2^2*l_4*sin(phi_4)*(l_5 - l_1*cos(phi_1) + l_4*cos(phi_4)))/(2*(4*l_2^2*(l_1*sin(phi_1) - l_4*sin(phi_4))^2 - ((l_1*sin(phi_1) - l_4*sin(phi_4))^2 + (l_5 - l_1*cos(phi_1) + l_4*cos(phi_4))^2 + l_2^2 - l_3^2)^2 + 4*l_2^2*(l_5 - l_1*cos(phi_1) + l_4*cos(phi_4))^2)^(1/2)) - 2*l_2*l_4*cos(phi_4))/((l_1*sin(phi_1) - l_4*sin(phi_4))^2 + (l_5 - l_1*cos(phi_1) + l_4*cos(phi_4))^2 + l_2^2 - l_3^2 + 2*l_2*(l_5 - l_1*cos(phi_1) + l_4*cos(phi_4))) - (((4*l_2^2*(l_1*sin(phi_1) - l_4*sin(phi_4))^2 - ((l_1*sin(phi_1) - l_4*sin(phi_4))^2 + (l_5 - l_1*cos(phi_1) + l_4*cos(phi_4))^2 + l_2^2 - l_3^2)^2 + 4*l_2^2*(l_5 - l_1*cos(phi_1) + l_4*cos(phi_4))^2)^(1/2) - 2*l_2*(l_1*sin(phi_1) - l_4*sin(phi_4)))*(2*l_2*l_4*sin(phi_4) + 2*l_4*cos(phi_4)*(l_1*sin(phi_1) - l_4*sin(phi_4)) + 2*l_4*sin(phi_4)*(l_5 - l_1*cos(phi_1) + l_4*cos(phi_4))))/((l_1*sin(phi_1) - l_4*sin(phi_4))^2 + (l_5 - l_1*cos(phi_1) + l_4*cos(phi_4))^2 + l_2^2 - l_3^2 + 2*l_2*(l_5 - l_1*cos(phi_1) + l_4*cos(phi_4)))^2))/(((l_2*sin(2*atan(((4*l_2^2*(l_1*sin(phi_1) - l_4*sin(phi_4))^2 - ((l_1*sin(phi_1) - l_4*sin(phi_4))^2 + (l_5 - l_1*cos(phi_1) + l_4*cos(phi_4))^2 + l_2^2 - l_3^2)^2 + 4*l_2^2*(l_5 - l_1*cos(phi_1) + l_4*cos(phi_4))^2)^(1/2) - 2*l_2*(l_1*sin(phi_1) - l_4*sin(phi_4)))/((l_1*sin(phi_1) - l_4*sin(phi_4))^2 + (l_5 - l_1*cos(phi_1) + l_4*cos(phi_4))^2 + l_2^2 - l_3^2 + 2*l_2*(l_5 - l_1*cos(phi_1) + l_4*cos(phi_4))))) + l_1*sin(phi_1))^2 + (l_2*cos(2*atan(((4*l_2^2*(l_1*sin(phi_1) - l_4*sin(phi_4))^2 - ((l_1*sin(phi_1) - l_4*sin(phi_4))^2 + (l_5 - l_1*cos(phi_1) + l_4*cos(phi_4))^2 + l_2^2 - l_3^2)^2 + 4*l_2^2*(l_5 - l_1*cos(phi_1) + l_4*cos(phi_4))^2)^(1/2) - 2*l_2*(l_1*sin(phi_1) - l_4*sin(phi_4)))/((l_1*sin(phi_1) - l_4*sin(phi_4))^2 + (l_5 - l_1*cos(phi_1) + l_4*cos(phi_4))^2 + l_2^2 - l_3^2 + 2*l_2*(l_5 - l_1*cos(phi_1) + l_4*cos(phi_4))))) - l_5/2 + l_1*cos(phi_1))^2)^(1/2)*(((4*l_2^2*(l_1*sin(phi_1) - l_4*sin(phi_4))^2 - ((l_1*sin(phi_1) - l_4*sin(phi_4))^2 + (l_5 - l_1*cos(phi_1) + l_4*cos(phi_4))^2 + l_2^2 - l_3^2)^2 + 4*l_2^2*(l_5 - l_1*cos(phi_1) + l_4*cos(phi_4))^2)^(1/2) - 2*l_2*(l_1*sin(phi_1) - l_4*sin(phi_4)))^2/((l_1*sin(phi_1) - l_4*sin(phi_4))^2 + (l_5 - l_1*cos(phi_1) + l_4*cos(phi_4))^2 + l_2^2 - l_3^2 + 2*l_2*(l_5 - l_1*cos(phi_1) + l_4*cos(phi_4)))^2 + 1)))/(1 - (l_2*cos(2*atan(((4*l_2^2*(l_1*sin(phi_1) - l_4*sin(phi_4))^2 - ((l_1*sin(phi_1) - l_4*sin(phi_4))^2 + (l_5 - l_1*cos(phi_1) + l_4*cos(phi_4))^2 + l_2^2 - l_3^2)^2 + 4*l_2^2*(l_5 - l_1*cos(phi_1) + l_4*cos(phi_4))^2)^(1/2) - 2*l_2*(l_1*sin(phi_1) - l_4*sin(phi_4)))/((l_1*sin(phi_1) - l_4*sin(phi_4))^2 + (l_5 - l_1*cos(phi_1) + l_4*cos(phi_4))^2 + l_2^2 - l_3^2 + 2*l_2*(l_5 - l_1*cos(phi_1) + l_4*cos(phi_4))))) - l_5/2 + l_1*cos(phi_1))^2/((l_2*sin(2*atan(((4*l_2^2*(l_1*sin(phi_1) - l_4*sin(phi_4))^2 - ((l_1*sin(phi_1) - l_4*sin(phi_4))^2 + (l_5 - l_1*cos(phi_1) + l_4*cos(phi_4))^2 + l_2^2 - l_3^2)^2 + 4*l_2^2*(l_5 - l_1*cos(phi_1) + l_4*cos(phi_4))^2)^(1/2) - 2*l_2*(l_1*sin(phi_1) - l_4*sin(phi_4)))/((l_1*sin(phi_1) - l_4*sin(phi_4))^2 + (l_5 - l_1*cos(phi_1) + l_4*cos(phi_4))^2 + l_2^2 - l_3^2 + 2*l_2*(l_5 - l_1*cos(phi_1) + l_4*cos(phi_4))))) + l_1*sin(phi_1))^2 + (l_2*cos(2*atan(((4*l_2^2*(l_1*sin(phi_1) - l_4*sin(phi_4))^2 - ((l_1*sin(phi_1) - l_4*sin(phi_4))^2 + (l_5 - l_1*cos(phi_1) + l_4*cos(phi_4))^2 + l_2^2 - l_3^2)^2 + 4*l_2^2*(l_5 - l_1*cos(phi_1) + l_4*cos(phi_4))^2)^(1/2) - 2*l_2*(l_1*sin(phi_1) - l_4*sin(phi_4)))/((l_1*sin(phi_1) - l_4*sin(phi_4))^2 + (l_5 - l_1*cos(phi_1) + l_4*cos(phi_4))^2 + l_2^2 - l_3^2 + 2*l_2*(l_5 - l_1*cos(phi_1) + l_4*cos(phi_4))))) - l_5/2 + l_1*cos(phi_1))^2))^(1/2);
J_T=[J11,J21;J12,J22];
J_Tinv=inv(J_T);
F=J_Tinv(1,1)*T1+J_Tinv(1,2)*T2;
Tp=J_Tinv(2,1)*T1+J_Tinv(2,2)*T2;
P=F*cos(theta)+Tp*sin(theta)/L_0;
F_N=P+m_w*g+m_w*a_w;
